simulink model "FuelCellBoostConverter"  (R2026b)
settings: Solver=VariableStepAuto
undefined symbols (not defined in the file): CtrlFcDcDcVoltCmd, PlntDCDCMass, PlntFcBusBarDiodeR
libraries: autolibdcdc x2, autolibutils x1, autolibsharedcommon x1
settings Model: ModifiedByFormat=The MathWorks, Inc.  Creator=The MathWorks, Inc.  LastModifiedBy=The MathWorks, Inc.
settings OptimizationCC: ReuseModelBlockBuffer=off

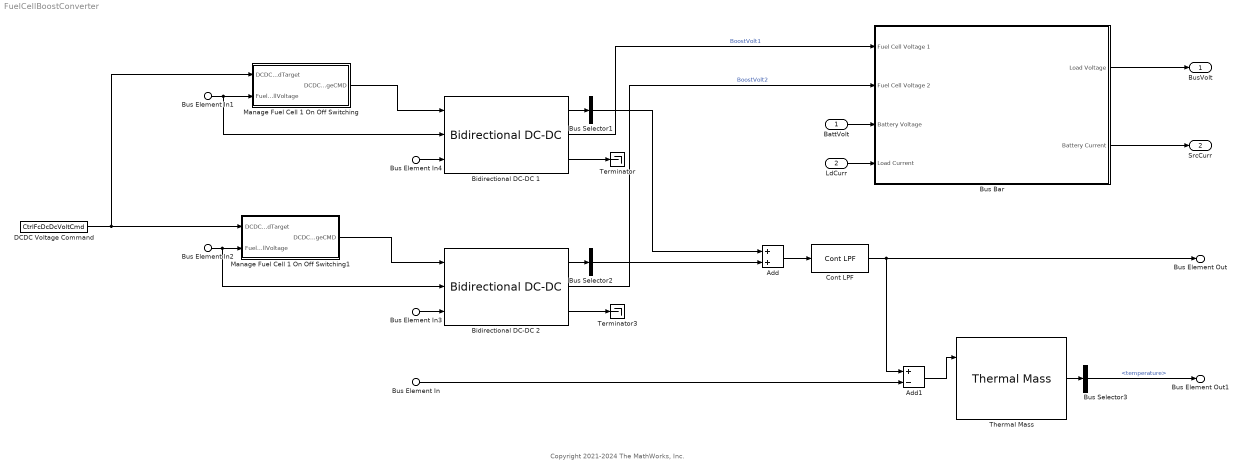
== system FuelCellBoostConverter ==
  note: Copyright 2021-2024 The MathWorks, Inc.
  BattVolt : Inport
  LdCurr : Inport  Port=2
  Bus Element In : Inport  Port=3  PortName=Thermal  Element=Qpwre
  Bus Element In1 : Inport  Port=4  PortName=FuelCell  Element=FuelCellVolt1
  Bus Element In2 : Inport  Port=4  PortName=FuelCell  Element=FuelCellVolt2
  Bus Element In3 : Inport  Port=4  PortName=FuelCell  Element=FuelCellCurr2
  Bus Element In4 : Inport  Port=4  PortName=FuelCell  Element=FuelCellCurr1
  Add : Sum
  Add1 : Sum  Inputs=+-
  Bidirectional DC-DC 1 : autolibdcdc/Bidirectional DC-DC  Tc=0.001  Vinit=650  Plimit=100000  param_loss=Single efficiency measurement  eff=PlntFcDcDcEff  v_loss_bp=[0 200 400 600 800 1000]  i_loss_bp=[0 25 50 75 100]  losses_table=[100 100 100 100 100;100 150 200 250 300;100 200 300 400 500;100 250 400 550 700;100 300 500 700 900;100 350 600 850 1100]  v_eff_bp=[200 400 600 800 1000]  i_eff_bp=[25 50 75 100]  efficiency_table=[96.2 98.1 98.7 99;98.1 99 99.4 99.5;98.7 99.4 99.6 99.7;99 99.5 99.7 99.8;99.2 99.6 99.7 99.8]  x_v_bp=[-1000 -800 -600 -400 -200 200 400 600 800 1000]  x_i_bp=[-100 -75 -50 -25 25 50 75 100]  x_losses_mat=[200.400801603196 225.67703109328 200.803212851408 201.612903225806 199.999999999997 200 225 200;160.320641282556 180.541624874624 201.005025125625 202.020202020203 200 200 180 160;180.541624874624 180.722891566267 181.086519114686 197.568389057748 194.999999999999 179.999999999997 180 180;201.005025125625 181.086519114686 202.020202020203 193.67991845056 190 200 179.999999999997 200;202.020202020203 197.568389057748 193.67991845056 197.505197505197 190 190 194.999999999999 200;200 194.999999999999 190 190 197.505197505197 193.67991845056 197.568389057748 202.020202020203;200 179.999999999997 200 190 193.67991845056 202.020202020203 181.086519114686 201.005025125625;180 180 179.999999999997 194.999999999999 197.568389057748 181.086519114686 180.722891566267 180.541624874624;160 180 200 200 202.020202020203 201.005025125625 180.541624874624 160.320641282556;200 225 200 199.999999999997 201.612903225806 200.803212851408 225.67703109328 200.400801603196]  RefBlkName='autolibdcdc/Bidirectional DC-DC'  CalLossMapData={'BaseCageProjectFileName','';'BaseMbcProjectFileName','';'TaskName','Calibrate Inverter Loss Map';'ChildTasks',{{'DataName','';'TaskName','Import Loss Data'},{'TaskName','Generate Response Models'},{'TaskName','Generate Calibration'},{'TaskName','Update Block Parameters'}}}
  Bidirectional DC-DC 2 : autolibdcdc/Bidirectional DC-DC  Tc=0.001  Vinit=650  Plimit=100000  param_loss=Single efficiency measurement  eff=PlntFcDcDcEff  v_loss_bp=[0 200 400 600 800 1000]  i_loss_bp=[0 25 50 75 100]  losses_table=[100 100 100 100 100;100 150 200 250 300;100 200 300 400 500;100 250 400 550 700;100 300 500 700 900;100 350 600 850 1100]  v_eff_bp=[200 400 600 800 1000]  i_eff_bp=[25 50 75 100]  efficiency_table=[96.2 98.1 98.7 99;98.1 99 99.4 99.5;98.7 99.4 99.6 99.7;99 99.5 99.7 99.8;99.2 99.6 99.7 99.8]  x_v_bp=[-1000 -800 -600 -400 -200 200 400 600 800 1000]  x_i_bp=[-100 -75 -50 -25 25 50 75 100]  x_losses_mat=[200.400801603196 225.67703109328 200.803212851408 201.612903225806 199.999999999997 200 225 200;160.320641282556 180.541624874624 201.005025125625 202.020202020203 200 200 180 160;180.541624874624 180.722891566267 181.086519114686 197.568389057748 194.999999999999 179.999999999997 180 180;201.005025125625 181.086519114686 202.020202020203 193.67991845056 190 200 179.999999999997 200;202.020202020203 197.568389057748 193.67991845056 197.505197505197 190 190 194.999999999999 200;200 194.999999999999 190 190 197.505197505197 193.67991845056 197.568389057748 202.020202020203;200 179.999999999997 200 190 193.67991845056 202.020202020203 181.086519114686 201.005025125625;180 180 179.999999999997 194.999999999999 197.568389057748 181.086519114686 180.722891566267 180.541624874624;160 180 200 200 202.020202020203 201.005025125625 180.541624874624 160.320641282556;200 225 200 199.999999999997 201.612903225806 200.803212851408 225.67703109328 200.400801603196]  RefBlkName='autolibdcdc/Bidirectional DC-DC'  CalLossMapData={'BaseCageProjectFileName','';'BaseMbcProjectFileName','';'TaskName','Calibrate Inverter Loss Map';'ChildTasks',{{'DataName','';'TaskName','Import Loss Data'},{'TaskName','Generate Response Models'},{'TaskName','Generate Calibration'},{'TaskName','Update Block Parameters'}}}
  Bus Selector1 : BusSelector  OutputSignals=PwrLoss  OutputAsBus=on
  Bus Selector2 : BusSelector  OutputSignals=PwrLoss  OutputAsBus=on
  Bus Selector3 : BusSelector  OutputSignals=temperature
  Bus Bar : Subsystem
  Cont LPF : autolibutils/Cont LPF  wc=1  AbsoluteTolerance=auto  aMode=6
  DCDC Voltage Command : Constant  Value=CtrlFcDcDcVoltCmd
  Manage Fuel Cell 1 On Off Switching : Subsystem
  Manage Fuel Cell 1 On Off Switching1 : Subsystem
  Terminator : Terminator
  Terminator3 : Terminator
  Thermal Mass : autolibsharedcommon/Thermal Mass  Mass=PlntDCDCMass  Cp=795
  BusVolt : Outport  VectorParamsAs1DForOutWhenUnconnected=off
  SrcCurr : Outport  Port=2  VectorParamsAs1DForOutWhenUnconnected=off
  Bus Element Out : Outport  Port=3  PortName=DCDC  Element=PwrELoss
  Bus Element Out1 : Outport  Port=3  PortName=DCDC  Element=PwrETemp
  wires:
  Bidirectional DC-DC 1/1 -> Bus Selector1/1
  Bus Bar/1(Load Voltage) -> BusVolt/1
  Bus Selector1/1 -> Add/1
  Cont LPF/1 -> Bus Element Out/1, Add1/1
  Bus Element In/1 -> Add1/2
  Thermal Mass/1 -> Bus Selector3/1
  Bus Selector3/1 -> Bus Element Out1/1  "<temperature>"
  Bus Bar/2(Battery Current) -> SrcCurr/1
  Bidirectional DC-DC 2/2 -> Bus Bar/2(Fuel Cell Voltage 2)  "BoostVolt2"
  Bidirectional DC-DC 1/2 -> Bus Bar/1(Fuel Cell Voltage 1)  "BoostVolt1"
  Bidirectional DC-DC 2/1 -> Bus Selector2/1
  Bidirectional DC-DC 1/3 -> Terminator/1
  Bidirectional DC-DC 2/3 -> Terminator3/1
  Add/1 -> Cont LPF/1
  Bus Selector2/1 -> Add/2
  LdCurr/1 -> Bus Bar/4(Load Current)
  BattVolt/1 -> Bus Bar/3(Battery Voltage)
  Bus Element In3/1 -> Bidirectional DC-DC 2/3
  Bus Element In4/1 -> Bidirectional DC-DC 1/3
  Add1/1 -> Thermal Mass/1
  Manage Fuel Cell 1 On Off Switching/1(DCDCVoltageCMD) -> Bidirectional DC-DC 1/1
  DCDC Voltage Command/1 -> Manage Fuel Cell 1 On Off Switching1/1(DCDCVoltageCmdTarget), Manage Fuel Cell 1 On Off Switching/1(DCDCVoltageCmdTarget)
  Bus Element In1/1 -> Manage Fuel Cell 1 On Off Switching/2(FuelCellVoltage), Bidirectional DC-DC 1/2
  Manage Fuel Cell 1 On Off Switching1/1(DCDCVoltageCMD) -> Bidirectional DC-DC 2/1
  Bus Element In2/1 -> Manage Fuel Cell 1 On Off Switching1/2(FuelCellVoltage), Bidirectional DC-DC 2/2

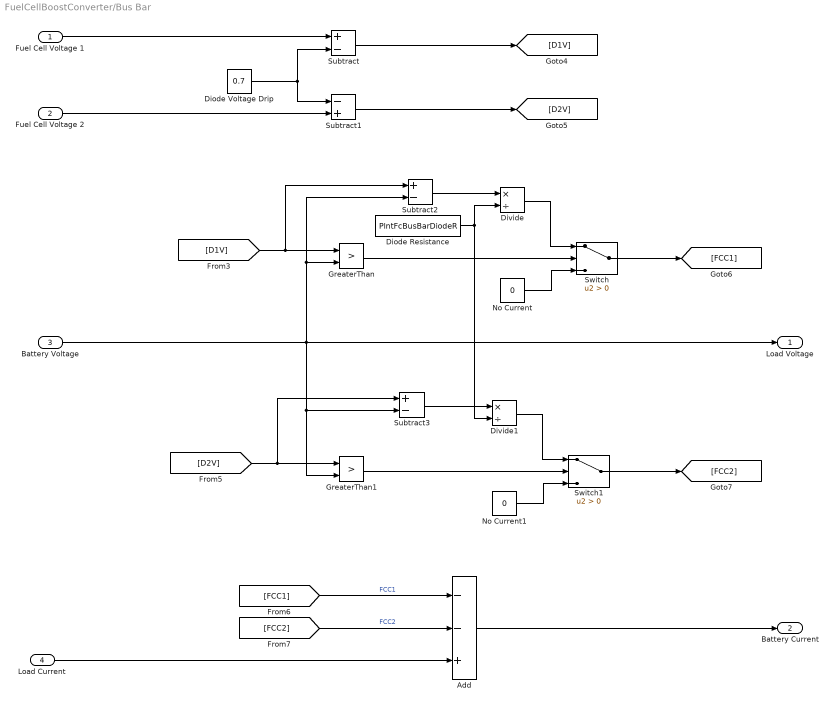
== system FuelCellBoostConverter/Bus Bar ==
  Fuel Cell Voltage 1 : Inport
  Fuel Cell Voltage 2 : Inport  Port=2
  Battery Voltage : Inport  Port=3
  Load Current : Inport  Port=4
  Add : Sum  Inputs=--+
  Diode Resistance : Constant  Value=PlntFcBusBarDiodeR
  Diode Voltage Drip : Constant  Value=0.7
  Divide : Product  Inputs=*/
  Divide1 : Product  Inputs=*/
  GreaterThan : RelationalOperator  Operator=>  OutDataTypeStr=boolean  RndMeth=Simplest  InputSameDT=off
  GreaterThan1 : RelationalOperator  Operator=>  OutDataTypeStr=boolean  RndMeth=Simplest  InputSameDT=off
  No Current : Constant  Value=0
  No Current1 : Constant  Value=0
  Subtract : Sum  Inputs=+-
  Subtract1 : Sum  Inputs=-+
  Subtract2 : Sum  Inputs=+-
  Subtract3 : Sum  Inputs=+-
  Switch : Switch  Criteria=u2 > Threshold  ZeroCross=off  SaturateOnIntegerOverflow=off  InputSameDT=off
  Switch1 : Switch  Criteria=u2 > Threshold  ZeroCross=off  SaturateOnIntegerOverflow=off  InputSameDT=off
  Load Voltage : Outport
  Battery Current : Outport  Port=2
  wires:
  Add/1 -> Battery Current/1
  [FCC2] -> Add/2  "FCC2"
  [FCC1] -> Add/1  "FCC1"
  Load Current/1 -> Add/3
  No Current/1 -> Switch/3
  Battery Voltage/1 -> Load Voltage/1, Subtract3/2, GreaterThan1/2, GreaterThan/2, Subtract2/2
  [D1V] -> GreaterThan/1, Subtract2/1
  Fuel Cell Voltage 2/1 -> Subtract1/2
  Diode Voltage Drip/1 -> Subtract/2, Subtract1/1
  Subtract1/1 -> [D2V]
  No Current1/1 -> Switch1/3
  Subtract3/1 -> Divide1/1
  GreaterThan/1 -> Switch/2
  Diode Resistance/1 -> Divide1/2, Divide/2
  Subtract2/1 -> Divide/1
  Divide/1 -> Switch/1
  GreaterThan1/1 -> Switch1/2
  Subtract/1 -> [D1V]
  Divide1/1 -> Switch1/1
  Switch/1 -> [FCC1]
  Switch1/1 -> [FCC2]
  [D2V] -> Subtract3/1, GreaterThan1/1
  Fuel Cell Voltage 1/1 -> Subtract/1

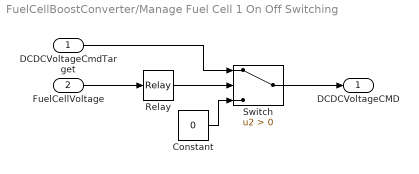
== system FuelCellBoostConverter/Manage Fuel Cell 1 On Off Switching ==
  DCDCVoltageCmdTarget : Inport
  FuelCellVoltage : Inport  Port=2
  Constant : Constant  Value=0
  Relay : Relay
  Switch : Switch  Criteria=u2 > Threshold  ZeroCross=off  SaturateOnIntegerOverflow=off  InputSameDT=off
  DCDCVoltageCMD : Outport
  wires:
  FuelCellVoltage/1 -> Relay/1
  Relay/1 -> Switch/2
  DCDCVoltageCmdTarget/1 -> Switch/1
  Constant/1 -> Switch/3
  Switch/1 -> DCDCVoltageCMD/1

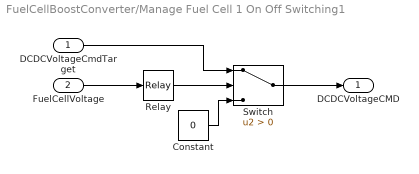
== system FuelCellBoostConverter/Manage Fuel Cell 1 On Off Switching1 ==
  DCDCVoltageCmdTarget : Inport
  FuelCellVoltage : Inport  Port=2
  Constant : Constant  Value=0
  Relay : Relay
  Switch : Switch  Criteria=u2 > Threshold  ZeroCross=off  SaturateOnIntegerOverflow=off  InputSameDT=off
  DCDCVoltageCMD : Outport
  wires:
  Switch/1 -> DCDCVoltageCMD/1
  Constant/1 -> Switch/3
  DCDCVoltageCmdTarget/1 -> Switch/1
  Relay/1 -> Switch/2
  FuelCellVoltage/1 -> Relay/1
